simulink model "slexPowerWindowSystemModel"  (R2014b)
settings: Solver=ode23  StartTime=0  StopTime=10  RelTol=1e-3
Description:
  | Main Power Window Model
settings Model: ModifiedByFormat=The MathWorks Inc.  Creator=The MathWorks Inc.  LastModifiedBy=The MathWorks Inc.
settings SolverCC: InsertRTBMode=Always
settings DataIOCC: SaveFormat=StructureWithTime  InspectSignalLogs=on  SignalLoggingName=sigsOut
settings OptimizationCC: ExpressionDepthLimit=2147483647
settings DebuggingCC: ArrayBoundsChecking=warning  UnderspecifiedInitializationDetection=Classic  MergeDetectMultiDrivingBlocksExec=none  SolverPrmCheckMsg=none  SigSpecEnsureSampleTimeMsg=none  ParameterPrecisionLossMsg=none  StateNameClashWarn=warning
settings ModelReferenceCC: ModelReferencePassRootInputsByReference=off
settings SimMechanicsCC: WarnOnRedundantConstraints=off

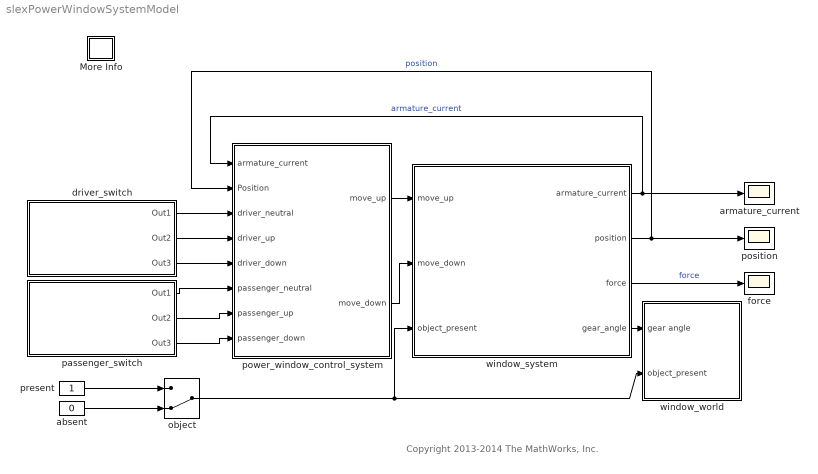
== system slexPowerWindowSystemModel ==
  note: Copyright 2013-2014 The MathWorks, Inc.
  More Info : Subsystem
      settings: OpenFcn=showdemo('slexPowerWindowScript')
      mask Display: disp('?')
  absent : Constant  Value=0  OutDataTypeStr=boolean
  armature_current : Scope
      settings: YMin=-15  YMax=15  SaveName=ScopeData2
  driver_switch : Subsystem  Variant=on
  force : Scope
      settings: YMin=-175  YMax=75  SaveName=ScopeData4
  object : ManualSwitch  CurrentSetting=0
  passenger_switch : Subsystem  Variant=on
  position : Scope
      settings: TimeRange=10  YMin=-0.5  YMax=0.5
  power_window_control_system : Subsystem
  present : Constant  OutDataTypeStr=boolean
  window_system : Subsystem  Variant=on
  window_world : Subsystem  LoadFcn=|  Variant=on
      | if license('test','virtual_reality_toolbox') & exist('slexPowerWindowMechWindow.wrl','file')
      |      SL3DBlock = [gcs '/window_world/Simulink_3D_Animation View/VR Sink'];
      |      vrmfunc('FnOpen', get_param(SL3DBlock,'handle'));
      | end
  wires:
  passenger_switch/1(Out1) -> power_window_control_system/6(passenger_neutral)
  passenger_switch/2(Out2) -> power_window_control_system/7(passenger_up)
  driver_switch/3(Out3) -> power_window_control_system/5(driver_down)
  driver_switch/2(Out2) -> power_window_control_system/4(driver_up)
  driver_switch/1(Out1) -> power_window_control_system/3(driver_neutral)
  power_window_control_system/1(move_up) -> window_system/1(move_up)
  power_window_control_system/2(move_down) -> window_system/2(move_down)
  window_system/1(armature_current) -> power_window_control_system/1(armature_current), armature_current/1  "armature_current"
  window_system/4(gear_angle) -> window_world/1(gear angle)
  window_system/3(force) -> force/1  "force"
  present/1 -> object/1
  absent/1 -> object/2
  window_system/2(position) -> power_window_control_system/2(Position), position/1  "position"
  object/1 -> window_system/3(object_present), window_world/2(object_present)
  passenger_switch/3(Out3) -> power_window_control_system/8(passenger_down)

== system slexPowerWindowSystemModel/More Info ==

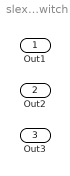
== system slexPowerWindowSystemModel/driver_switch ==
  Out1 : Outport
  Out2 : Outport  Port=2
  Out3 : Outport  Port=3

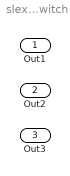
== system slexPowerWindowSystemModel/passenger_switch ==
  Out1 : Outport
  Out2 : Outport  Port=2
  Out3 : Outport  Port=3

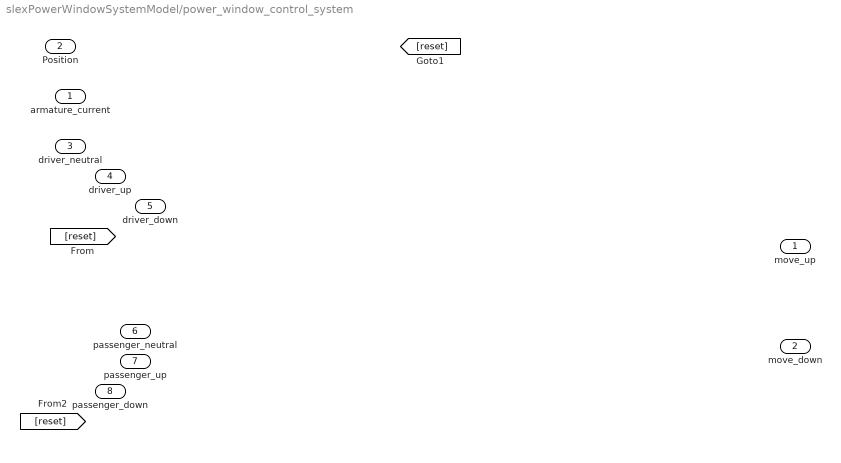
== system slexPowerWindowSystemModel/power_window_control_system ==
  armature_current : Inport
  Position : Inport  Port=2
  driver_neutral : Inport  Port=3
  driver_up : Inport  Port=4
  driver_down : Inport  Port=5
  passenger_neutral : Inport  Port=6
  passenger_up : Inport  Port=7
  passenger_down : Inport  Port=8
  move_up : Outport
  move_down : Outport  Port=2

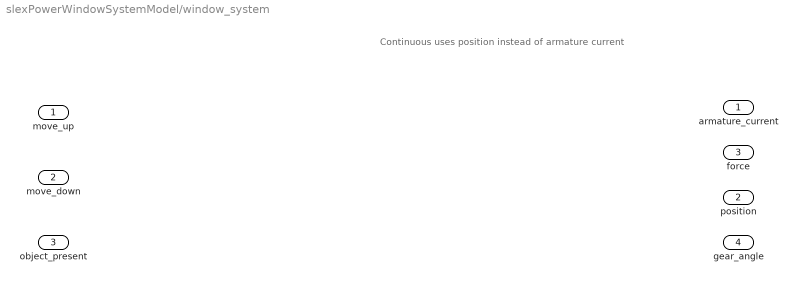
== system slexPowerWindowSystemModel/window_system ==
  note: Continuous uses position instead of armature current
  move_up : Inport
  move_down : Inport  Port=2
  object_present : Inport  Port=3
  armature_current : Outport
  position : Outport  Port=2
  force : Outport  Port=3
  gear_angle : Outport  Port=4

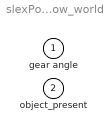
== system slexPowerWindowSystemModel/window_world ==
  gear angle : Inport
  object_present : Inport  Port=2
